simulink model "advances_pid"  (R2018b)
settings: Solver=FixedStepDiscrete  StartTime=0.0  StopTime=10  FixedStep=0.001  RelTol=0.01
undefined symbols (not defined in the file or in its folder): DiscIntNeverNeededParam
settings Model: Creator=kika  LastModifiedBy=kika

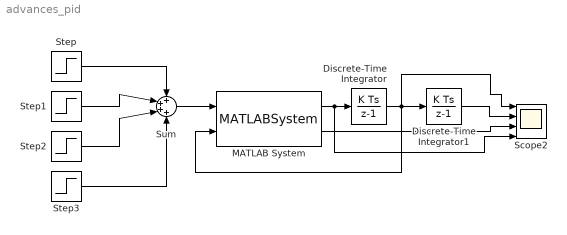
== system advances_pid ==
  Discrete-Time Integrator : DiscreteIntegrator  SampleTime=-1  ICPrevOutput=DiscIntNeverNeededParam  ICPrevScaledInput=DiscIntNeverNeededParam
  Discrete-Time Integrator1 : DiscreteIntegrator  SampleTime=-1  ICPrevOutput=DiscIntNeverNeededParam  ICPrevScaledInput=DiscIntNeverNeededParam
  MATLAB System : MATLABSystem  System=PID  dt=0.001  feedback_nature=1  kp=10  ki=2  kd=0  u_max=2  u_min=-2  input_clip=true  output_clip=true  ramp=true  velocity_profile_type=0  x0=0  v0=0  a0=0  x_range=[ -pi, pi ]  v_max=3  a_max=3  j_max=0  antiwindup=false  kt=1  SimulateUsing=Code generation
      mask Type: PID
      mask Display:
      | disp('PID');
      | port_label('input',1,'in_des');
      | port_label('input',2,'in_state');
      | port_label('output',1,'out');
      | port_label('output',2,'e');
  Scope2 : Scope  NumInputPorts=4
  Step : Step  SampleTime=0
  Step1 : Step  Time=2  After=1.5  SampleTime=0
  Step2 : Step  Time=4  After=-1  SampleTime=0
  Step3 : Step  Time=6  After=-2  SampleTime=0
  Sum : Sum  Inputs=++++
  wires:
  Sum/1 -> MATLAB System/1
  MATLAB System/1 -> Scope2/4, Discrete-Time Integrator/1
  Discrete-Time Integrator/1 -> MATLAB System/2, Scope2/1, Discrete-Time Integrator1/1
  Discrete-Time Integrator1/1 -> Scope2/2
  MATLAB System/2 -> Scope2/3
  Step/1 -> Sum/1
  Step1/1 -> Sum/2
  Step2/1 -> Sum/3
  Step3/1 -> Sum/4
